simulink model "testing_DM_hby"  (R2023b)
settings: Solver=FixedStepDiscrete  StartTime=0.0  StopTime=inf  FixedStep=0.003  RelTol=1e-3
InitFcn:
  | run('/home/uonaim/matlab_ws/FOOT/joint_calibration.m');
undefined symbols (not defined in the file or in its folder): CAL
libraries: ros2lib x12
(part 1 of 2)
settings Model: Creator=root  LastModifiedBy=root
settings OptimizationCC: EnhancedBackFolding=on  PassReuseOutputArgsAs=Individual arguments  ZeroExternalMemoryAtStartup=off  ZeroInternalMemoryAtStartup=off  MaxStackSize=64  OptimizeBlockOrder=speed  DifferentSizesBufferReuse=on  OptimizationCustomize=off  EfficientTunableParamExpr=on
settings DebuggingCC: ParameterTunabilityLossMsg=error
settings HardwareCC: ProdBitPerLong=64  ProdHWDeviceType=Intel->x86-64 (Linux 64)
settings SFSimCC: MATLABDynamicMemAlloc=off
settings RTWCC: Description=Embedded Coder  SystemTargetFile=ert.tlc  HardwareBoard=Robot Operating System 2 (ROS 2)  TLCOptions="-aInlineSetEventsForThisBaseRateFcn=TLC_FALSE -aSuppressMultiTaskScheduler=TLC_FALSE  -aRateBasedStepFcn=0"  TemplateMakefile=ert_default_tmf  Toolchain=Colcon Tools  TargetLang=C++
settings CodeAppCC: ForceParamTrailComments=on  IgnoreCustomStorageClasses=off  OperatorAnnotations=on  SimulinkDataObjDesc=on  SFDataObjDesc=on  InsertBlockDesc=on
settings ERTTargetCC: CodeInterfacePackaging=C++ class  SupportContinuousTime=on  RootIOFormat=Structure reference

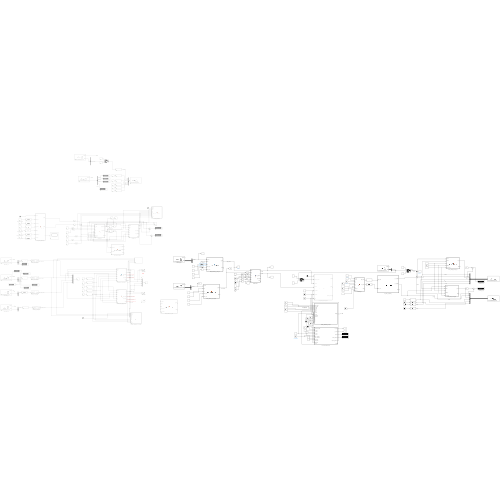
[thumbnail: Simulink's stored preview of the top-level diagram]
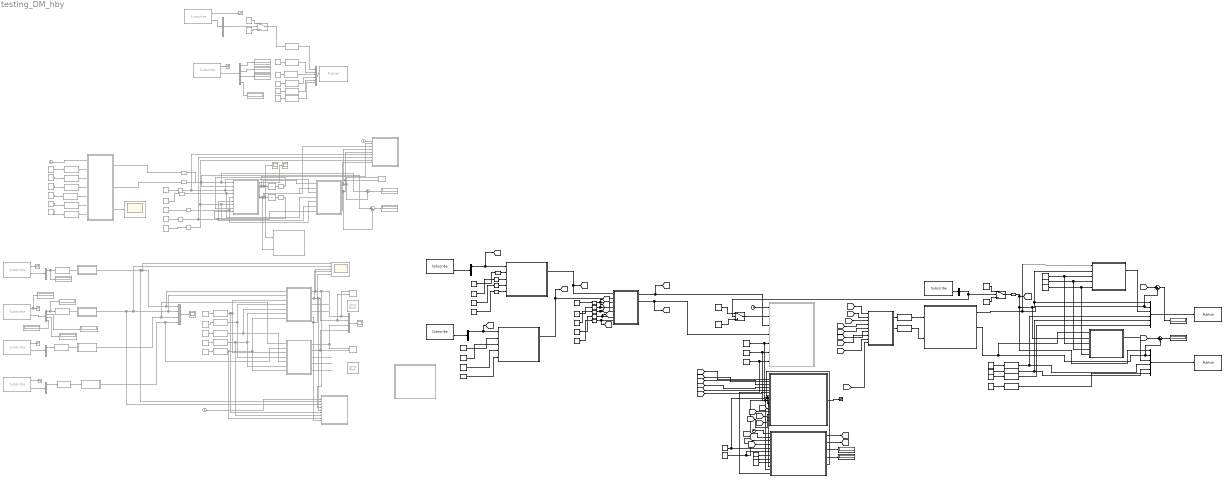
== system testing_DM_hby ==
  note: single(20)
  A : Constant  Value=-0.24
  Alpha Memory : UnitDelay  Commented=on  InitialCondition=CAL.qj0_LA  SampleTime=-1  HasFrameUpgradeWarning=on
  B : Constant  Value=0.24
  Beta Memory : UnitDelay  Commented=on  InitialCondition=CAL.qj0_LB  SampleTime=-1  HasFrameUpgradeWarning=on
  Bus Creator : BusCreator  Commented=on  Inputs=6  OutDataTypeStr=Bus: SL_Bus_custom_msgs_WriteDmMotorMITControl  NonVirtualBus=on
      settings: InheritFromInputs=off
  Bus Creator1 : BusCreator  Inputs=6  OutDataTypeStr=Bus: SL_Bus_custom_msgs_WriteDmMotorMITControl  NonVirtualBus=on
  Bus Creator2 : BusCreator  Inputs=6  OutDataTypeStr=Bus: SL_Bus_custom_msgs_WriteDmMotorMITControl  NonVirtualBus=on
  Bus Selector : BusSelector  Commented=on  OutputSignals=position,velocity,torque,online
  Bus Selector1 : BusSelector  Commented=on  OutputSignals=right_switch
  Bus Selector2 : BusSelector  Commented=on  OutputSignals=position,velocity,torque
  Bus Selector3 : BusSelector  Commented=on  OutputSignals=position,velocity,torque
  Bus Selector4 : BusSelector  Commented=on  OutputSignals=position,velocity,torque,overload
  Bus Selector5 : BusSelector  Commented=on  OutputSignals=position,velocity,torque
  Bus Selector6 : BusSelector  OutputSignals=position,velocity,torque
  Bus Selector7 : BusSelector  OutputSignals=position,velocity,torque
  Bus Selector8 : BusSelector  OutputSignals=right_switch
  Clock : Clock  Commented=on
  Clock1 : Clock  Commented=on
  Clock2 : Clock  Commented=on
  Clock3 : Clock
  Clock4 : Clock
  Constant : Constant  Commented=on
  Constant{1,4..6} (4 alike) : Constant  Commented=on  Value=0
  Constant10 : Constant  Value=CAL.ratio_LA
  Constant11 : Constant  Value=CAL.ratio_LB
  Constant12 : Constant  Value=CAL.qm0_LB
  Constant13 : Constant  Value=CAL.qj0_LB
  Constant14 : Constant  Value=CAL.sign_LB
  Constant15 : Constant  Value=true  OutDataTypeStr=boolean
  Constant16 : Constant  Value=single(0.05)
  Constant17 : Constant  Value=single(0.02)
  Constant18 : Constant  Value=single(20)
  Constant19 : Constant  Value=single(0.035)
  Constant2 : Constant  Commented=on  Value=0.9
  Constant20 : Constant  Value=single(0.1)
  Constant21 : Constant  Value=single(5.0)
  Constant22 : Constant  Value=single(0.003)
  Constant23 : Constant
  Constant24 : Constant  Value=0
  Constant25 : Constant  Value=single(0.5)
  Constant26 : Constant  Value=3.3
  Constant27 : Constant  Value=0.09
  Constant29 : Constant  Value=single(0.003)
  Constant3 : Constant  Commented=on  Value=0.1
  Constant30 : Constant  Value=single(8.0)
  Constant31 : Constant  Value=single(0.5)
  Constant32 : Constant  Value=false  OutDataTypeStr=boolean
  Constant7 : Constant  Value=CAL.qm0_LA
  Constant8 : Constant  Value=CAL.qj0_LA
  Constant9 : Constant  Value=CAL.sign_LA
  Data Type Conversion : DataTypeConversion  Commented=on  OutDataTypeStr=uint8  SaturateOnIntegerOverflow=off  RndMeth=Floor
  Data Type Conversion{1..29} (29 alike) : DataTypeConversion  Commented=on  OutDataTypeStr=single  SaturateOnIntegerOverflow=off  RndMeth=Floor
  Data Type Conversion{30..40,42,46..48} (15 alike) : DataTypeConversion  OutDataTypeStr=single  SaturateOnIntegerOverflow=off  RndMeth=Floor
  Data Type Conversion41 : DataTypeConversion  OutDataTypeStr=uint8  SaturateOnIntegerOverflow=off  RndMeth=Floor
  Display{,1..11} (12 alike) : Display  Commented=on
  Display12 : Display
  Display13 : Display
  FiveBar_Animation : MATLAB Function  Commented=on  TreatAsAtomicUnit=on
  FiveBar_Animation_Compare : MATLAB Function  TreatAsAtomicUnit=on
  FiveBar_Animation_Left_Actual : MATLAB Function  Commented=on  TreatAsAtomicUnit=on
  FiveBar_FK : MATLAB Function  Commented=on  TreatAsAtomicUnit=on
  FiveBar_FK1 : MATLAB Function  TreatAsAtomicUnit=on
  FiveBar_FK_Left_Actual : MATLAB Function  Commented=on  TreatAsAtomicUnit=on
  FiveBar_FK_Right_Actual : MATLAB Function  Commented=on  TreatAsAtomicUnit=on
  FiveBar_IK : MATLAB Function  Commented=on  TreatAsAtomicUnit=on
  FiveBar_IK1 : MATLAB Function  TreatAsAtomicUnit=on
  Foot_Home_Then_Sine : MATLAB Function  TreatAsAtomicUnit=on
  Foot_Sine_Trajectory : MATLAB Function  Commented=on  TreatAsAtomicUnit=on
  Foot_Sine_Trajectory_HW : MATLAB Function  Commented=on  TreatAsAtomicUnit=on
  L{1,4,6,9} (4 alike) : Constant  Commented=on  Value=0.0804
  L10 : Constant  Commented=on  Value=0.07
  L11 : Constant  Value=0.0804
  L12 : Constant  Value=0.12
  L13 : Constant  Value=0.12
  L14 : Constant  Value=0.0804
  L15 : Constant  Value=0.07
  L{2..3,7..8} (4 alike) : Constant  Commented=on  Value=0.12
  L5 : Constant  Commented=on  Value=0.07
  Lamp : LampBlock  Commented=on  LabelPosition=Hide  Icon=Check3
  Lamp1 : LampBlock  Commented=on  LabelPosition=Hide
  Left_Joint_To_Motor : MATLAB Function  Commented=on  TreatAsAtomicUnit=on
  Left_Joint_To_Motor_L : MATLAB Function  TreatAsAtomicUnit=on
  Motor_Position_To_Joint : MATLAB Function  Commented=on  TreatAsAtomicUnit=on
  Motor_Position_To_Joint_LA : MATLAB Function  TreatAsAtomicUnit=on
  Motor_Position_To_Joint_LB : MATLAB Function  TreatAsAtomicUnit=on
  Motor_Target_Velocity_LA : MATLAB Function  TreatAsAtomicUnit=on
  Motor_Target_Velocity_LB : MATLAB Function  TreatAsAtomicUnit=on
  Motor_To_Joint_LA : Subsystem  Commented=on
  Motor_To_Joint_LB : Subsystem  Commented=on
  Motor_To_Joint_RA : Subsystem  Commented=on
  Motor_To_Joint_RB : Subsystem  Commented=on
  Mux : Mux  Commented=on
  Mux1 : Mux  Commented=on
  Publish : ros2lib/Publish  Commented=on  topicSource=Select from ROS network  topic=/ecat/sn2228252/app4/write  messageType=custom_msgs/WriteDmMotorMITControl  QOSHistory=Keep last  QOSDepth=1  QOSReliability=Best effort  QOSDurability=Volatile
  Publish1 : ros2lib/Publish  topicSource=Select from ROS network  topic=/ecat/sn2228252/app2/write  messageType=custom_msgs/WriteDmMotorMITControl  QOSHistory=Keep last  QOSDepth=1  QOSReliability=Best effort  QOSDurability=Volatile
  Publish2 : ros2lib/Publish  topicSource=Select from ROS network  topic=/ecat/sn2228252/app3/write  messageType=custom_msgs/WriteDmMotorMITControl  QOSHistory=Keep last  QOSDepth=1  QOSReliability=Best effort  QOSDurability=Volatile
  Scope{,1..4} (5 alike) : Scope  Commented=on
  Scope5 : Scope  Commented=on  NumInputPorts=5
  Subscribe : ros2lib/Subscribe  Commented=on  topicSource=Select from ROS network  topic=/ecat/sn2228252/app4/read  messageType=custom_msgs/ReadDmMotor  sampleTime=-1  QOSHistory=Keep last  QOSDepth=1  QOSReliability=Best effort  QOSDurability=Volatile
  Subscribe1 : ros2lib/Subscribe  Commented=on  topicSource=Select from ROS network  topic=/ecat/sn2228252/app1/read  messageType=custom_msgs/ReadDJIRC  sampleTime=-1  QOSHistory=Keep last  QOSDepth=1  QOSReliability=Best effort  QOSDurability=Volatile
  Subscribe2 : ros2lib/Subscribe  Commented=on  topicSource=Select from ROS network  topic=/ecat/sn2228252/app3/read  messageType=custom_msgs/ReadDmMotor  sampleTime=-1  QOSHistory=Keep last  QOSDepth=1  QOSReliability=Best effort  QOSDurability=Volatile
  Subscribe3 : ros2lib/Subscribe  topicSource=Select from ROS network  topic=/ecat/sn2228252/app3/read  messageType=custom_msgs/ReadDmMotor  sampleTime=-1  QOSHistory=Keep last  QOSDepth=1  QOSReliability=Best effort  QOSDurability=Volatile
  Subscribe4 : ros2lib/Subscribe  topicSource=Select from ROS network  topic=/ecat/sn2228252/app1/read  messageType=custom_msgs/ReadDJIRC  sampleTime=-1  QOSHistory=Keep last  QOSDepth=1  QOSReliability=Best effort  QOSDurability=Volatile
  Subscribe_LA : ros2lib/Subscribe  Commented=on  topicSource=Select from ROS network  topic=/ecat/sn2228252/app2/read  messageType=custom_msgs/ReadDmMotor  sampleTime=-1  QOSHistory=Keep last  QOSDepth=1  QOSReliability=Best effort  QOSDurability=Volatile
  Subscribe_LA1 : ros2lib/Subscribe  topicSource=Select from ROS network  topic=/ecat/sn2228252/app2/read  messageType=custom_msgs/ReadDmMotor  sampleTime=-1  QOSHistory=Keep last  QOSDepth=1  QOSReliability=Best effort  QOSDurability=Volatile
  Subscribe_RA : ros2lib/Subscribe  Commented=on  topicSource=Select from ROS network  topic=/ecat/sn2228252/app5/read  messageType=custom_msgs/ReadDmMotor  sampleTime=-1  QOSHistory=Keep last  QOSDepth=1  QOSReliability=Best effort  QOSDurability=Volatile
  Subscribe_RB : ros2lib/Subscribe  Commented=on  topicSource=Select from ROS network  topic=/ecat/sn2228252/app6/read  messageType=custom_msgs/ReadDmMotor  sampleTime=-1  QOSHistory=Keep last  QOSDepth=1  QOSReliability=Best effort  QOSDurability=Volatile
  Sum : Sum  Inputs=|+-
  Sum1 : Sum  Inputs=|+-
  Switch : Switch  Commented=on  Criteria=u2 > Threshold  Threshold=2  SaturateOnIntegerOverflow=off  InputSameDT=off
  Switch1 : Switch  Criteria=u2 > Threshold  Threshold=2  SaturateOnIntegerOverflow=off  InputSameDT=off
  Switch2 : Switch  Criteria=u2 > Threshold  Threshold=2  SaturateOnIntegerOverflow=off  InputSameDT=off
  Terminator{,1..5} (6 alike) : Terminator  Commented=on
  Terminator6 : Terminator
  Trajectory_Amplitude : Constant  Commented=on  Value=0.01
  Trajectory_Enable : Constant  Commented=on
  Trajectory_Period : Constant  Commented=on  Value=10
  Trajectory_Width : Constant  Commented=on  Value=0.02
  X Error : Sum  Commented=on  Inputs=|+-
  XY Graph : Record  Commented=on  FileSettingsInternal="{\"entries\":[{\"content\":{\"excelSettings\":{\"content\":{},\"type\":\"Streamout.ExcelSettings\"}},\"type\":\"Streamout.FileSettingStorage\",\"uuid\":\"\"}],\"packageUris\":[\"http:\\/\\/schema.mathworks.com\\/mf0\\/streamout_blocks\\/R2020a\"],\"version\":\"1.0\"}"  Layout=[1 1]  SignalsInternal="{\"entries\":[{\"content\":{\"signals\":[{\"content\":{\"blockPath\":[],\"dimensions\":[1],\"domain\":\"\",\"lineColor\":\"#a2142f\",\"port\":1,\"sid\":[\"\"],\"signalID\":1,\"signalName\":\"FiveBar_FK:1\"},\"type\":\"RecordBlkView.Signal\",\"uuid\":\"\"},{\"content\":{\"blockPath\":[],\"dimensions\":[1],\"domain\":\"\",\"lineColor\":\"#139fff\",\"port\":2,\"sid\":[\"\"],\"signalID\":2,\"signalName\":\"FiveBar_FK:2\"},\"type\":\"RecordBlkView.Signal\",\"uuid\":\"\"}]},\"type\":\"RecordBlkView.InputSignals\",\"uuid\":\"\"}],\"packageUris\":[\"http:\\/\\/schema.mathworks.com\\/mf0\\/streamout_blocks\\/R2020a\"],\"version\":\"1.0\"}"  VisualizationBindings="{\"xyplotplugin\":{\"info\":[{\"series\":[],\"subplotID\":1}]}}"  CompatibilityTag=XY
  XY Graph1 : Record  Commented=on  FileSettingsInternal="{\"entries\":[{\"content\":{\"excelSettings\":{\"content\":{},\"type\":\"Streamout.ExcelSettings\"}},\"type\":\"Streamout.FileSettingStorage\",\"uuid\":\"\"}],\"packageUris\":[\"http:\\/\\/schema.mathworks.com\\/mf0\\/streamout_blocks\\/R2020a\"],\"version\":\"1.0\"}"  Layout=[1 1]  SignalsInternal="{\"entries\":[{\"content\":{},\"type\":\"RecordBlkView.InputSignals\",\"uuid\":\"\"}],\"packageUris\":[\"http:\\/\\/schema.mathworks.com\\/mf0\\/streamout_blocks\\/R2020a\"],\"version\":\"1.0\"}"  VisualizationBindings="{\"xyplotplugin\":{\"info\":[{\"series\":[],\"subplotID\":1}]}}"  CompatibilityTag=XY
  XY Graph2 : Record  Commented=on  FileSettingsInternal="{\"entries\":[{\"content\":{\"excelSettings\":{\"content\":{},\"type\":\"Streamout.ExcelSettings\"}},\"type\":\"Streamout.FileSettingStorage\",\"uuid\":\"\"}],\"packageUris\":[\"http:\\/\\/schema.mathworks.com\\/mf0\\/streamout_blocks\\/R2020a\"],\"version\":\"1.0\"}"  Layout=[1 1]  SignalsInternal="{\"entries\":[{\"content\":{},\"type\":\"RecordBlkView.InputSignals\",\"uuid\":\"\"}],\"packageUris\":[\"http:\\/\\/schema.mathworks.com\\/mf0\\/streamout_blocks\\/R2020a\"],\"version\":\"1.0\"}"  VisualizationBindings="{\"xyplotplugin\":{\"info\":[{\"series\":[],\"subplotID\":1}]}}"  CompatibilityTag=XY
  X_Center : Constant  Commented=on  Value=0.035
  Y Error : Sum  Commented=on  Inputs=|+-
  Y_Center : Constant  Commented=on  Value=0.12
  position_err_A : Display
  position_err_B : Display
  wires:
  Subscribe/1 -> Terminator/1
  Subscribe/2 -> Bus Selector/1
  Bus Selector/4 -> Display/1  "<online>"
  Bus Selector/1 -> Display3/1  "<position>"
  Bus Selector/2 -> Display1/1  "<velocity>"
  Bus Selector/3 -> Display2/1  "<torque>"
  Bus Creator/1 -> Publish/1
  Constant1/1 -> Data Type Conversion1/1
  Constant3/1 -> Data Type Conversion4/1
  Constant4/1 -> Data Type Conversion3/1
  Constant2/1 -> Data Type Conversion2/1
  Data Type Conversion/1 -> Bus Creator/1  "enable"
  Data Type Conversion1/1 -> Bus Creator/2  "p_des"
  Data Type Conversion2/1 -> Bus Creator/3  "v_des"
  Data Type Conversion3/1 -> Bus Creator/4  "kp"
  Data Type Conversion4/1 -> Bus Creator/5  "kd"
  Constant5/1 -> Data Type Conversion5/1
  Data Type Conversion5/1 -> Bus Creator/6  "torque"
  Constant/1 -> Switch/1
  Switch/1 -> Data Type Conversion/1
  Subscribe1/1 -> Terminator1/1
  Subscribe1/2 -> Bus Selector1/1
  Bus Selector1/1 -> Switch/2  "<right_switch>"
  Constant6/1 -> Switch/3
  FiveBar_IK/1(alpha_cmd) -> FiveBar_Animation/2(alpha), FiveBar_FK/1(alpha), Left_Joint_To_Motor/1(alpha_cmd), Scope1/1, Alpha Memory/1
  Alpha Memory/1 -> Data Type Conversion6/1
  FiveBar_IK/2(beta_cmd) -> Left_Joint_To_Motor/2(beta_cmd), FiveBar_Animation/3(beta), Beta Memory/1, FiveBar_FK/2(beta), Scope2/1
  Beta Memory/1 -> Data Type Conversion7/1
  L2/1 -> Data Type Conversion11/1
  L3/1 -> Data Type Conversion12/1
  L4/1 -> Data Type Conversion13/1
  L5/1 -> Data Type Conversion14/1
  L1/1 -> Data Type Conversion10/1
  FiveBar_FK/1(x) -> FiveBar_Animation/4(xB), X Error/2, XY Graph/1
  FiveBar_FK/2(y) -> XY Graph/2, FiveBar_Animation/5(yB), Y Error/2
  X Error/1 -> Display4/1
  Y Error/1 -> Display5/1
  Data Type Conversion6/1 -> FiveBar_IK/8(alpha_ref)
  Data Type Conversion7/1 -> FiveBar_IK/9(beta_ref)
  Data Type Conversion8/1 -> X Error/1, FiveBar_IK/1(x_cmd)
  Data Type Conversion9/1 -> Y Error/1, FiveBar_IK/2(y_cmd)
  Data Type Conversion10/1 -> FiveBar_Animation/6(L1), FiveBar_FK/3(L1), FiveBar_IK/3(L1)
  Data Type Conversion11/1 -> FiveBar_FK/4(L2), FiveBar_IK/4(L2)
  Data Type Conversion12/1 -> FiveBar_IK/5(L3), FiveBar_FK/5(L3)
  Data Type Conversion13/1 -> FiveBar_Animation/7(L4), FiveBar_IK/6(L4), FiveBar_FK/6(L4)
  Data Type Conversion14/1 -> FiveBar_Animation/8(L5), FiveBar_FK/7(L5), FiveBar_IK/7(L5)
  FiveBar_FK/5(valid) -> FiveBar_Animation/9(valid)
  Trajectory_Enable/1 -> Data Type Conversion16/1
  Clock/1 -> Foot_Sine_Trajectory/1(time_in)
  Data Type Conversion16/1 -> Foot_Sine_Trajectory/2(enable_in)
  X_Center/1 -> Data Type Conversion17/1
  Y_Center/1 -> Data Type Conversion18/1
  Data Type Conversion17/1 -> Foot_Sine_Trajectory/3(x_center_in)
  Data Type Conversion18/1 -> Foot_Sine_Trajectory/4(y_center_in)
  Trajectory_Width/1 -> Data Type Conversion19/1
  Data Type Conversion19/1 -> Foot_Sine_Trajectory/5(width_in)
  Trajectory_Amplitude/1 -> Data Type Conversion20/1
  Data Type Conversion20/1 -> Foot_Sine_Trajectory/6(amplitude_in)
  Trajectory_Period/1 -> Data Type Conversion21/1
  Data Type Conversion21/1 -> Foot_Sine_Trajectory/7(period_in)
  Foot_Sine_Trajectory/1(x_cmd) -> Data Type Conversion8/1
  Foot_Sine_Trajectory/2(y_cmd) -> Data Type Conversion9/1
  Foot_Sine_Trajectory/3(s) -> Scope/1
  Clock1/1 -> FiveBar_Animation/1(time_in)
  Subscribe_LA/2 -> Bus Selector2/1
  Bus Selector2/1 -> Display11/1, Data Type Conversion15/1  "<position>"
  Subscribe_LA/1 -> Terminator2/1
  Subscribe_RA/2 -> Bus Selector3/1
  Subscribe_RB/2 -> Bus Selector5/1
  Subscribe2/2 -> Bus Selector4/1
  Subscribe2/1 -> Display6/1, Terminator3/1
  Subscribe_RA/1 -> Terminator4/1
  Subscribe_RB/1 -> Terminator5/1
  Bus Selector3/1 -> Data Type Conversion23/1  "<position>"
  Bus Selector5/1 -> Data Type Conversion24/1  "<position>"
  Data Type Conversion15/1 -> Motor_To_Joint_LA/1(q_motor)
  Data Type Conversion22/1 -> Motor_To_Joint_LB/1(q_motor)
  Data Type Conversion23/1 -> Motor_To_Joint_RA/1(q_motor)
  Data Type Conversion24/1 -> Motor_To_Joint_RB/1(q_motor)
  Motor_To_Joint_LA/1(q_joint) -> FiveBar_Animation_Left_Actual/2(alpha), Scope5/1, FiveBar_FK_Left_Actual/1(alpha), Mux/1  "alpha_left_meas"
  Motor_To_Joint_LB/1(q_joint) -> FiveBar_Animation_Left_Actual/3(beta), Scope5/2, FiveBar_FK_Left_Actual/2(beta), Mux/2  "beta_left_meas"
  Motor_To_Joint_RA/1(q_joint) -> FiveBar_FK_Right_Actual/1(alpha), Mux/3  "alpha_right_meas"
  Motor_To_Joint_RB/1(q_joint) -> FiveBar_FK_Right_Actual/2(beta), Mux/4  "beta_right_meas"
  Mux/1 -> Scope3/1
  L6/1 -> Data Type Conversion25/1
  Data Type Conversion25/1 -> FiveBar_Animation_Left_Actual/6(L1), FiveBar_FK_Right_Actual/3(L1), FiveBar_FK_Left_Actual/3(L1)
  L7/1 -> Data Type Conversion26/1
  Data Type Conversion26/1 -> FiveBar_FK_Left_Actual/4(L2), FiveBar_FK_Right_Actual/4(L2)
  L8/1 -> Data Type Conversion27/1
  Data Type Conversion27/1 -> FiveBar_FK_Right_Actual/5(L3), FiveBar_FK_Left_Actual/5(L3)
  L9/1 -> Data Type Conversion28/1
  L10/1 -> Data Type Conversion29/1
  Data Type Conversion29/1 -> FiveBar_Animation_Left_Actual/8(L5), FiveBar_FK_Left_Actual/7(L5), FiveBar_FK_Right_Actual/7(L5)
  FiveBar_FK_Left_Actual/1(x) -> Scope5/3, FiveBar_Animation_Left_Actual/4(xB), XY Graph1/1, Mux1/1  "x_left_actual"
  FiveBar_FK_Left_Actual/2(y) -> Scope5/4, FiveBar_Animation_Left_Actual/5(yB), XY Graph1/2, Mux1/2  "y_left_actual"
  FiveBar_FK_Left_Actual/3(leg_length) -> ?  "leg_length_left_actual"
  FiveBar_FK_Left_Actual/4(leg_angle) -> ?  "leg_angle_left_actual"
  FiveBar_FK_Left_Actual/5(valid) -> Scope5/5, FiveBar_Animation_Left_Actual/9(valid)  "fk_valid_left"
  FiveBar_FK_Right_Actual/1(x) -> XY Graph2/1, Mux1/3  "x_right_actual"
  FiveBar_FK_Right_Actual/2(y) -> XY Graph2/2, Mux1/4  "y_right_actual"
  FiveBar_FK_Right_Actual/3(leg_length) -> ?  "leg_length_right_actual"
  FiveBar_FK_Right_Actual/4(leg_angle) -> ?  "leg_angle_right_actual"
  FiveBar_FK_Right_Actual/5(valid) -> ?  "fk_valid_right"
  Mux1/1 -> Scope4/1
  Clock2/1 -> FiveBar_Animation_Left_Actual/1(time_in)
  Data Type Conversion28/1 -> FiveBar_Animation_Left_Actual/7(L4), FiveBar_FK_Right_Actual/6(L4), FiveBar_FK_Left_Actual/6(L4)
  Bus Selector4/1 -> Data Type Conversion22/1, Display7/1  "<position>"
  Bus Selector4/2 -> Display8/1  "<velocity>"
  Bus Selector4/3 -> Display9/1  "<torque>"
  Bus Selector4/4 -> Display10/1  "<overload>"
  Subscribe_LA1/2 -> Bus Selector6/1
  Bus Selector6/1 -> [actual_pos_A], Motor_Position_To_Joint_LA/1(q_motor)  "<position>"
  Constant7/1 -> Data Type Conversion35/1
  Constant8/1 -> Data Type Conversion36/1
  Constant9/1 -> Data Type Conversion37/1
  Constant10/1 -> Data Type Conversion38/1
  Subscribe3/2 -> Bus Selector7/1
  Bus Selector7/1 -> [actual_pos_B], Motor_Position_To_Joint_LB/1(q_motor)  "<position>"
  Constant13/1 -> Motor_Position_To_Joint_LB/3(qj0)
  Constant12/1 -> Motor_Position_To_Joint_LB/2(qm0)
  Constant14/1 -> Motor_Position_To_Joint_LB/4(motor_sign)
  Constant11/1 -> Motor_Position_To_Joint_LB/5(motor_ratio)
  Motor_Position_To_Joint_LA/1(q_joint) -> [alpha_actual], FiveBar_FK1/1(alpha)  "alpha_actual"
  Motor_Position_To_Joint_LB/1(q_joint) -> FiveBar_FK1/2(beta), [beta_actual]  "beta_actual"
  L15/1 -> Data Type Conversion34/1
  L14/1 -> Data Type Conversion33/1
  L11/1 -> Data Type Conversion30/1
  L12/1 -> Data Type Conversion31/1
  L13/1 -> Data Type Conversion32/1
  Data Type Conversion30/1 -> [L1], FiveBar_FK1/3(L1)
  Data Type Conversion31/1 -> [L2], FiveBar_FK1/4(L2)
  Data Type Conversion33/1 -> [L4], FiveBar_FK1/6(L4)
  Data Type Conversion34/1 -> [L5], FiveBar_FK1/7(L5)
  Data Type Conversion35/1 -> Motor_Position_To_Joint_LA/2(qm0)
  Data Type Conversion36/1 -> Motor_Position_To_Joint_LA/3(qj0)
  Data Type Conversion37/1 -> Motor_Position_To_Joint_LA/4(motor_sign)
  Data Type Conversion38/1 -> Motor_Position_To_Joint_LA/5(motor_ratio)
  FiveBar_FK1/1(x) -> [x_actual], Foot_Sine_Trajectory_HW/3(x_actual)  "x_actual"
  FiveBar_FK1/2(y) -> [y_actual], Foot_Sine_Trajectory_HW/4(y_actual)  "y_actual"
  Clock3/1 -> Foot_Sine_Trajectory_HW/1(t)
  Constant16/1 -> Foot_Home_Then_Sine/10(path_width), FiveBar_Animation_Compare/10(path_width), Foot_Sine_Trajectory_HW/5(path_width)
  Constant17/1 -> Foot_Home_Then_Sine/11(amplitude), FiveBar_Animation_Compare/11(amplitude), Foot_Sine_Trajectory_HW/6(amplitude)
  Constant18/1 -> Foot_Home_Then_Sine/12(period), Foot_Sine_Trajectory_HW/7(period)
  [L1] -> FiveBar_IK1/3(L1)
  [L2] -> FiveBar_IK1/4(L2)
  [L3] -> FiveBar_IK1/5(L3)
  [L4] -> FiveBar_IK1/6(L4)
  [L5] -> FiveBar_IK1/7(L5)
  Data Type Conversion32/1 -> [L3], FiveBar_FK1/5(L3)
  FiveBar_IK1/1(alpha_cmd) -> Data Type Conversion39/1
  FiveBar_IK1/2(beta_cmd) -> Data Type Conversion40/1
  [alpha_actual] -> FiveBar_IK1/8(alpha_ref)
  [beta_actual] -> FiveBar_IK1/9(beta_ref)
  Data Type Conversion39/1 -> Left_Joint_To_Motor_L/1(alpha_cmd)
  Data Type Conversion40/1 -> Left_Joint_To_Motor_L/2(beta_cmd)
  Left_Joint_To_Motor_L/1(p_LA_target) -> Motor_Target_Velocity_LA/1(p_cmd), Sum/2, Bus Creator1/2  "p_des"
  Bus Creator1/1 -> Publish1/1
  Constant23/1 -> Switch1/1
  Constant24/1 -> Switch1/3
  Subscribe4/2 -> Bus Selector8/1
  Bus Selector8/1 -> Switch2/2, Switch1/2  "<right_switch>"
  Switch1/1 -> Data Type Conversion41/1  "enable"
  Bus Creator2/1 -> Publish2/1
  Constant26/1 -> Data Type Conversion46/1
  Constant27/1 -> Data Type Conversion47/1
  A/1 -> Data Type Conversion48/1
  Left_Joint_To_Motor_L/2(p_LB_target) -> Motor_Target_Velocity_LB/1(p_cmd), Sum1/2, Bus Creator2/2  "p_des"
  Data Type Conversion46/1 -> Bus Creator1/4, Bus Creator2/4  "kp"
  Data Type Conversion47/1 -> Bus Creator1/5, Bus Creator2/5  "kd"
  Data Type Conversion48/1 -> Bus Creator1/6  "torque"
  Constant29/1 -> Motor_Target_Velocity_LB/3(Ts), Motor_Target_Velocity_LA/3(Ts)
  Constant30/1 -> Motor_Target_Velocity_LB/4(cutoff_hz), Motor_Target_Velocity_LA/4(cutoff_hz)
  Constant31/1 -> Motor_Target_Velocity_LB/5(max_velocity), Motor_Target_Velocity_LA/5(max_velocity)
  Motor_Target_Velocity_LA/1(v_des) -> Bus Creator1/3  "v_des"
  Motor_Target_Velocity_LB/1(v_des) -> Bus Creator2/3  "v_des"
  Switch2/1 -> Foot_Sine_Trajectory_HW/2(trajectory_enable)
  Constant15/1 -> Switch2/1
  Constant32/1 -> Switch2/3
  [alpha_actual] -> FiveBar_Animation_Compare/1(alpha_actual)
  [beta_actual] -> FiveBar_Animation_Compare/2(beta_actual)
  [x_actual] -> FiveBar_Animation_Compare/3(x_actual)
  [y_actual] -> FiveBar_Animation_Compare/4(y_actual)
  [x_cmd2] -> FiveBar_Animation_Compare/5(x_cmd)
  [y_cmd2] -> FiveBar_Animation_Compare/6(y_cmd)
  [L2] -> FiveBar_Animation_Compare/13(L2)
  [L1] -> FiveBar_Animation_Compare/12(L1)
  [L3] -> FiveBar_Animation_Compare/14(L3)
  [L4] -> FiveBar_Animation_Compare/15(L4)
  [L5] -> FiveBar_Animation_Compare/16(L5)
  FiveBar_Animation_Compare/1(dummy) -> Terminator6/1
  Data Type Conversion41/1 -> [enable], Bus Creator2/1, Motor_Target_Velocity_LB/2(enable), Motor_Target_Velocity_LA/2(enable), Bus Creator1/1  "enable"
  [x_actual] -> Foot_Home_Then_Sine/3(x_actual)
  Constant19/1 -> FiveBar_Animation_Compare/8(x_home), Foot_Home_Then_Sine/5(x_home)
  Clock4/1 -> Foot_Home_Then_Sine/1(t)
  [y_actual] -> Foot_Home_Then_Sine/4(y_actual)
  Constant21/1 -> Foot_Home_Then_Sine/7(home_duration)
  Constant20/1 -> FiveBar_Animation_Compare/9(y_home), Foot_Home_Then_Sine/6(y_home)
  [enable] -> Foot_Home_Then_Sine/2(sequence_enable)
  Constant22/1 -> Foot_Home_Then_Sine/8(home_tolerance)
  Constant25/1 -> Foot_Home_Then_Sine/9(settle_time)
  Foot_Home_Then_Sine/2(y_cmd) -> [y_cmd2]
  Foot_Home_Then_Sine/1(x_cmd) -> [x_cmd2]
  [x_cmd2] -> FiveBar_IK1/1(x_cmd)
  [y_cmd2] -> FiveBar_IK1/2(y_cmd)
  Foot_Home_Then_Sine/3(phase) -> Display12/1
  Foot_Home_Then_Sine/4(home_reached) -> Display13/1
  Foot_Home_Then_Sine/5(trajectory_active) -> FiveBar_Animation_Compare/7(phase)
  B/1 -> Data Type Conversion42/1
  Data Type Conversion42/1 -> Bus Creator2/6  "torque"
  [actual_pos_A] -> Sum/1
  Sum/1 -> position_err_A/1
  [actual_pos_B] -> Sum1/1
  Sum1/1 -> position_err_B/1

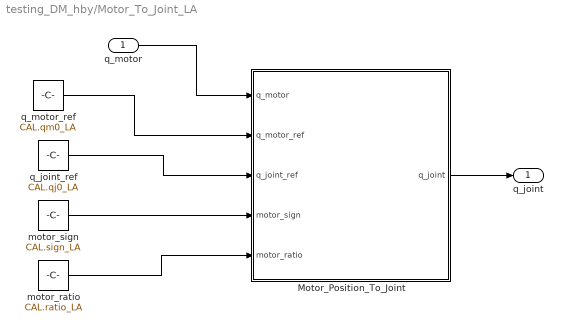
== system testing_DM_hby/Motor_To_Joint_LA ==
  q_motor : Inport
  Motor_Position_To_Joint : MATLAB Function  TreatAsAtomicUnit=on
  motor_ratio : Constant  Value=CAL.ratio_LA
  motor_sign : Constant  Value=CAL.sign_LA
  q_joint_ref : Constant  Value=CAL.qj0_LA
  q_motor_ref : Constant  Value=CAL.qm0_LA
  q_joint : Outport
  wires:
  q_motor/1 -> Motor_Position_To_Joint/1(q_motor)
  q_motor_ref/1 -> Motor_Position_To_Joint/2(q_motor_ref)
  q_joint_ref/1 -> Motor_Position_To_Joint/3(q_joint_ref)
  motor_sign/1 -> Motor_Position_To_Joint/4(motor_sign)
  motor_ratio/1 -> Motor_Position_To_Joint/5(motor_ratio)
  Motor_Position_To_Joint/1(q_joint) -> q_joint/1

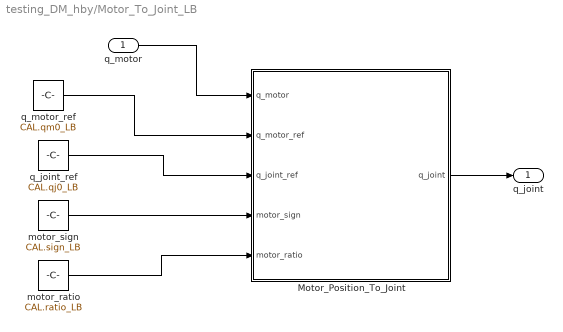
== system testing_DM_hby/Motor_To_Joint_LB ==
  q_motor : Inport
  Motor_Position_To_Joint : MATLAB Function  TreatAsAtomicUnit=on
  motor_ratio : Constant  Value=CAL.ratio_LB
  motor_sign : Constant  Value=CAL.sign_LB
  q_joint_ref : Constant  Value=CAL.qj0_LB
  q_motor_ref : Constant  Value=CAL.qm0_LB
  q_joint : Outport
  wires:
  q_motor/1 -> Motor_Position_To_Joint/1(q_motor)
  q_motor_ref/1 -> Motor_Position_To_Joint/2(q_motor_ref)
  q_joint_ref/1 -> Motor_Position_To_Joint/3(q_joint_ref)
  motor_sign/1 -> Motor_Position_To_Joint/4(motor_sign)
  motor_ratio/1 -> Motor_Position_To_Joint/5(motor_ratio)
  Motor_Position_To_Joint/1(q_joint) -> q_joint/1

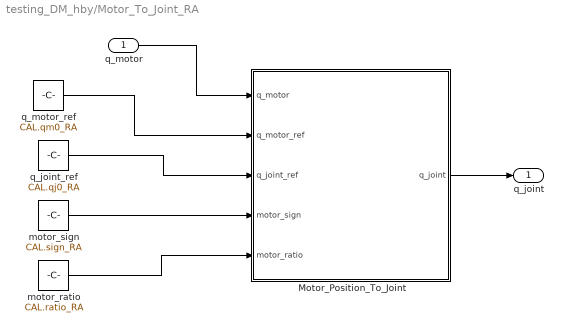
== system testing_DM_hby/Motor_To_Joint_RA ==
  q_motor : Inport
  Motor_Position_To_Joint : MATLAB Function  TreatAsAtomicUnit=on
  motor_ratio : Constant  Value=CAL.ratio_RA
  motor_sign : Constant  Value=CAL.sign_RA
  q_joint_ref : Constant  Value=CAL.qj0_RA
  q_motor_ref : Constant  Value=CAL.qm0_RA
  q_joint : Outport
  wires:
  q_motor/1 -> Motor_Position_To_Joint/1(q_motor)
  q_motor_ref/1 -> Motor_Position_To_Joint/2(q_motor_ref)
  q_joint_ref/1 -> Motor_Position_To_Joint/3(q_joint_ref)
  motor_sign/1 -> Motor_Position_To_Joint/4(motor_sign)
  motor_ratio/1 -> Motor_Position_To_Joint/5(motor_ratio)
  Motor_Position_To_Joint/1(q_joint) -> q_joint/1

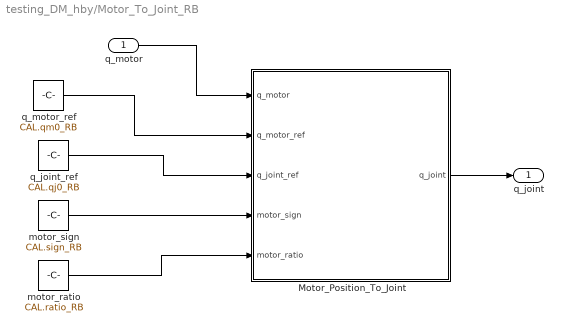
== system testing_DM_hby/Motor_To_Joint_RB ==
  q_motor : Inport
  Motor_Position_To_Joint : MATLAB Function  TreatAsAtomicUnit=on
  motor_ratio : Constant  Value=CAL.ratio_RB
  motor_sign : Constant  Value=CAL.sign_RB
  q_joint_ref : Constant  Value=CAL.qj0_RB
  q_motor_ref : Constant  Value=CAL.qm0_RB
  q_joint : Outport
  wires:
  q_motor/1 -> Motor_Position_To_Joint/1(q_motor)
  q_motor_ref/1 -> Motor_Position_To_Joint/2(q_motor_ref)
  q_joint_ref/1 -> Motor_Position_To_Joint/3(q_joint_ref)
  motor_sign/1 -> Motor_Position_To_Joint/4(motor_sign)
  motor_ratio/1 -> Motor_Position_To_Joint/5(motor_ratio)
  Motor_Position_To_Joint/1(q_joint) -> q_joint/1

== matlab function testing_DM_hby/Motor_To_Joint_LB/Motor_Position_To_Joint ==
  data: q_motor input; q_joint output; q_motor_ref input; q_joint_ref input; motor_sign input; motor_ratio input
function q_joint = motor_position_to_joint( ...
    q_motor, q_motor_ref, q_joint_ref, ...
    motor_sign, motor_ratio)
%#codegen
%
% 电机位置反馈转换为运动学关节角
%
% q_motor      当前电机位置反馈，rad
% q_motor_ref  标定参考姿态下的电机位置，rad
% q_joint_ref  标定参考姿态下的模型关节角，rad
% motor_sign   +1 或 -1
% motor_ratio  电机角变化/关节角变化

qm = single(q_motor);
qm0 = single(q_motor_ref);
qj0 = single(q_joint_ref);
sgn = single(motor_sign);
ratio = single(motor_ratio);

q_joint = qj0;

if abs(ratio) > single(1.0e-6)
    q_joint = qj0 + ...
        sgn * (qm - qm0) / ratio;
end

end

== matlab function testing_DM_hby/Motor_To_Joint_RA/Motor_Position_To_Joint ==
  data: q_motor input; q_joint output; q_motor_ref input; q_joint_ref input; motor_sign input; motor_ratio input
function q_joint = motor_position_to_joint( ...
    q_motor, q_motor_ref, q_joint_ref, ...
    motor_sign, motor_ratio)
%#codegen
%
% 电机位置反馈转换为运动学关节角
%
% q_motor      当前电机位置反馈，rad
% q_motor_ref  标定参考姿态下的电机位置，rad
% q_joint_ref  标定参考姿态下的模型关节角，rad
% motor_sign   +1 或 -1
% motor_ratio  电机角变化/关节角变化

qm = single(q_motor);
qm0 = single(q_motor_ref);
qj0 = single(q_joint_ref);
sgn = single(motor_sign);
ratio = single(motor_ratio);

q_joint = qj0;

if abs(ratio) > single(1.0e-6)
    q_joint = qj0 + ...
        sgn * (qm - qm0) / ratio;
end

end

== matlab function testing_DM_hby/Motor_To_Joint_RB/Motor_Position_To_Joint ==
  data: q_motor input; q_joint output; q_motor_ref input; q_joint_ref input; motor_sign input; motor_ratio input
function q_joint = motor_position_to_joint( ...
    q_motor, q_motor_ref, q_joint_ref, ...
    motor_sign, motor_ratio)
%#codegen
%
% 电机位置反馈转换为运动学关节角
%
% q_motor      当前电机位置反馈，rad
% q_motor_ref  标定参考姿态下的电机位置，rad
% q_joint_ref  标定参考姿态下的模型关节角，rad
% motor_sign   +1 或 -1
% motor_ratio  电机角变化/关节角变化

qm = single(q_motor);
qm0 = single(q_motor_ref);
qj0 = single(q_joint_ref);
sgn = single(motor_sign);
ratio = single(motor_ratio);

q_joint = qj0;

if abs(ratio) > single(1.0e-6)
    q_joint = qj0 + ...
        sgn * (qm - qm0) / ratio;
end

end

== matlab function testing_DM_hby/FiveBar_FK_Left_Actual ==
  data: x output; alpha input; y output; beta input; L1 input; L2 input; L3 input; L4 input; L5 input; leg_length output; leg_angle output; valid output
function [x, y, leg_length, leg_angle, valid] = ...
    fivebar_fk(alpha, beta, L1, L2, L3, L4, L5)
%#codegen
%
% 平面五连杆正运动学
%
% O = (0,0)
% D = (L5,0)
% x 向右为正
% y 向下为正
%
% 角度单位：rad
% 长度单位：m

x = single(0.0);
y = single(0.0);
leg_length = single(0.0);
leg_angle  = single(0.0);
valid = false;

eps_d = single(1.0e-6);

%% 两根主动杆末端

Ax = L1 * cos(alpha);
Ay = L1 * sin(alpha);

Cx = L5 + L4 * cos(beta);
Cy = L4 * sin(beta);

%% 求以 A、C 为圆心的两个圆交点

dx = Cx - Ax;
dy = Cy - Ay;

Dac = sqrt(dx * dx + dy * dy);

if Dac < eps_d
    return;
end

if Dac > (L2 + L3)
    return;
end

if Dac < abs(L2 - L3)
    return;
end

a = ...
    (L2 * L2 - L3 * L3 + Dac * Dac) / ...
    (single(2.0) * Dac);

h2 = L2 * L2 - a * a;

if h2 < single(-1.0e-7)
    return;
end

if h2 < single(0.0)
    h2 = single(0.0);
end

h = sqrt(h2);

ux = dx / Dac;
uy = dy / Dac;

Mx = Ax + a * ux;
My = Ay + a * uy;

% 两个可能的轮心位置
x1 = Mx - h * uy;
y1 = My + h * ux;

x2 = Mx + h * uy;
y2 = My - h * ux;

% y 向下为正，因此选下面的交点
if y1 >= y2
    x = x1;
    y = y1;
else
    x = x2;
    y = y2;
end

%% 虚拟腿长和虚拟腿角

center_x = L5 / single(2.0);

leg_x = x - center_x;
leg_y = y;

leg_length = sqrt(leg_x * leg_x + leg_y * leg_y);

% 竖直向下时 leg_angle = 0
leg_angle = atan2(leg_x, leg_y);

valid = true;

end

== matlab function testing_DM_hby/FiveBar_FK_Right_Actual ==
  data: x output; alpha input; y output; beta input; L1 input; L2 input; L3 input; L4 input; L5 input; leg_length output; leg_angle output; valid output
function [x, y, leg_length, leg_angle, valid] = ...
    fivebar_fk(alpha, beta, L1, L2, L3, L4, L5)
%#codegen
%
% 平面五连杆正运动学
%
% O = (0,0)
% D = (L5,0)
% x 向右为正
% y 向下为正
%
% 角度单位：rad
% 长度单位：m

x = single(0.0);
y = single(0.0);
leg_length = single(0.0);
leg_angle  = single(0.0);
valid = false;

eps_d = single(1.0e-6);

%% 两根主动杆末端

Ax = L1 * cos(alpha);
Ay = L1 * sin(alpha);

Cx = L5 + L4 * cos(beta);
Cy = L4 * sin(beta);

%% 求以 A、C 为圆心的两个圆交点

dx = Cx - Ax;
dy = Cy - Ay;

Dac = sqrt(dx * dx + dy * dy);

if Dac < eps_d
    return;
end

if Dac > (L2 + L3)
    return;
end

if Dac < abs(L2 - L3)
    return;
end

a = ...
    (L2 * L2 - L3 * L3 + Dac * Dac) / ...
    (single(2.0) * Dac);

h2 = L2 * L2 - a * a;

if h2 < single(-1.0e-7)
    return;
end

if h2 < single(0.0)
    h2 = single(0.0);
end

h = sqrt(h2);

ux = dx / Dac;
uy = dy / Dac;

Mx = Ax + a * ux;
My = Ay + a * uy;

% 两个可能的轮心位置
x1 = Mx - h * uy;
y1 = My + h * ux;

x2 = Mx + h * uy;
y2 = My - h * ux;

% y 向下为正，因此选下面的交点
if y1 >= y2
    x = x1;
    y = y1;
else
    x = x2;
    y = y2;
end

%% 虚拟腿长和虚拟腿角

center_x = L5 / single(2.0);

leg_x = x - center_x;
leg_y = y;

leg_length = sqrt(leg_x * leg_x + leg_y * leg_y);

% 竖直向下时 leg_angle = 0
leg_angle = atan2(leg_x, leg_y);

valid = true;

end

== matlab function testing_DM_hby/FiveBar_Animation_Left_Actual ==
  data: time_in input; alpha input; beta input; xB input; yB input; L1 input; L4 input; L5 input; valid input
function FiveBar_Animation( ...
    time_in, alpha, beta, xB, yB, L1, L4, L5, valid)
%#codegen

coder.extrinsic('fivebar_plot_smooth');

if coder.target('Sfun')

    fivebar_plot_smooth( ...
        double(time_in), ...
        double(alpha), ...
        double(beta), ...
        double(xB), ...
        double(yB), ...
        double(L1), ...
        double(L4), ...
        double(L5), ...
        logical(valid));

end

end

== matlab function testing_DM_hby/Motor_Position_To_Joint ==
  data: q_motor input; q_joint output; qm0 input; qj0 input; motor_sign input; motor_ratio input; valid output
function [q_joint, valid] = Motor_Position_To_Joint( ...
    q_motor, qm0, qj0, motor_sign, motor_ratio)
%#codegen
% 将电机反馈角度转换为五连杆主动关节角
%
% 标定关系：
% q_joint = qj0 + (q_motor - qm0) * motor_sign / motor_ratio

% 统一使用single，匹配ROS消息中的float32
q_motor    = single(q_motor);
qm0        = single(qm0);
qj0        = single(qj0);
motor_sign = single(motor_sign);
motor_ratio = single(motor_ratio);

% 默认输出
q_joint = qj0;
valid = false;

% 检查输入是否有效
if ~isfinite(q_motor) || ...
   ~isfinite(qm0) || ...
   ~isfinite(qj0) || ...
   ~isfinite(motor_sign) || ...
   ~isfinite(motor_ratio)
    return;
end

% 防止除以0
if abs(motor_ratio) < single(1.0e-6)
    return;
end

% 电机角转换为关节角
q_joint = qj0 + ...
    (q_motor - qm0) * motor_sign / motor_ratio;

valid = isfinite(q_joint);

end

== matlab function testing_DM_hby/Motor_Position_To_Joint_LA ==
  data: q_motor input; q_joint output; qm0 input; qj0 input; motor_sign input; motor_ratio input; valid output
function [q_joint, valid] = Motor_Position_To_Joint( ...
    q_motor, qm0, qj0, motor_sign, motor_ratio)
%#codegen
% 将电机反馈角度转换为五连杆主动关节角
%
% 标定关系：
% q_joint = qj0 + (q_motor - qm0) * motor_sign / motor_ratio

% 统一使用single，匹配ROS消息中的float32
q_motor    = single(q_motor);
qm0        = single(qm0);
qj0        = single(qj0);
motor_sign = single(motor_sign);
motor_ratio = single(motor_ratio);

% 默认输出
q_joint = qj0;
valid = false;

% 检查输入是否有效
if ~isfinite(q_motor) || ...
   ~isfinite(qm0) || ...
   ~isfinite(qj0) || ...
   ~isfinite(motor_sign) || ...
   ~isfinite(motor_ratio)
    return;
end

% 防止除以0
if abs(motor_ratio) < single(1.0e-6)
    return;
end

% 电机角转换为关节角
q_joint = qj0 + ...
    (q_motor - qm0) * motor_sign / motor_ratio;

valid = isfinite(q_joint);

end

== matlab function testing_DM_hby/Motor_Position_To_Joint_LB ==
  data: q_motor input; q_joint output; qm0 input; qj0 input; motor_sign input; motor_ratio input; valid output
function [q_joint, valid] = Motor_Position_To_Joint( ...
    q_motor, qm0, qj0, motor_sign, motor_ratio)
%#codegen
% 将电机反馈角度转换为五连杆主动关节角
%
% 标定关系：
% q_joint = qj0 + (q_motor - qm0) * motor_sign / motor_ratio

% 统一使用single，匹配ROS消息中的float32
q_motor    = single(q_motor);
qm0        = single(qm0);
qj0        = single(qj0);
motor_sign = single(motor_sign);
motor_ratio = single(motor_ratio);

% 默认输出
q_joint = qj0;
valid = false;

% 检查输入是否有效
if ~isfinite(q_motor) || ...
   ~isfinite(qm0) || ...
   ~isfinite(qj0) || ...
   ~isfinite(motor_sign) || ...
   ~isfinite(motor_ratio)
    return;
end

% 防止除以0
if abs(motor_ratio) < single(1.0e-6)
    return;
end

% 电机角转换为关节角
q_joint = qj0 + ...
    (q_motor - qm0) * motor_sign / motor_ratio;

valid = isfinite(q_joint);

end

== matlab function testing_DM_hby/FiveBar_FK1 ==
  data: x output; alpha input; y output; beta input; L1 input; L2 input; L3 input; L4 input; L5 input; leg_length output; leg_angle output; valid output
function [x, y, leg_length, leg_angle, valid] = ...
    fivebar_fk(alpha, beta, L1, L2, L3, L4, L5)
%#codegen
%
% 平面五连杆正运动学
%
% O = (0,0)
% D = (L5,0)
% x 向右为正
% y 向下为正
%
% 角度单位：rad
% 长度单位：m

x = single(0.0);
y = single(0.0);
leg_length = single(0.0);
leg_angle  = single(0.0);
valid = false;

eps_d = single(1.0e-6);

%% 两根主动杆末端

Ax = L1 * cos(alpha);
Ay = L1 * sin(alpha);

Cx = L5 + L4 * cos(beta);
Cy = L4 * sin(beta);

%% 求以 A、C 为圆心的两个圆交点

dx = Cx - Ax;
dy = Cy - Ay;

Dac = sqrt(dx * dx + dy * dy);

if Dac < eps_d
    return;
end

if Dac > (L2 + L3)
    return;
end

if Dac < abs(L2 - L3)
    return;
end

a = ...
    (L2 * L2 - L3 * L3 + Dac * Dac) / ...
    (single(2.0) * Dac);

h2 = L2 * L2 - a * a;

if h2 < single(-1.0e-7)
    return;
end

if h2 < single(0.0)
    h2 = single(0.0);
end

h = sqrt(h2);

ux = dx / Dac;
uy = dy / Dac;

Mx = Ax + a * ux;
My = Ay + a * uy;

% 两个可能的轮心位置
x1 = Mx - h * uy;
y1 = My + h * ux;

x2 = Mx + h * uy;
y2 = My - h * ux;

% y 向下为正，因此选下面的交点
if y1 >= y2
    x = x1;
    y = y1;
else
    x = x2;
    y = y2;
end

%% 虚拟腿长和虚拟腿角

center_x = L5 / single(2.0);

leg_x = x - center_x;
leg_y = y;

leg_length = sqrt(leg_x * leg_x + leg_y * leg_y);

% 竖直向下时 leg_angle = 0
leg_angle = atan2(leg_x, leg_y);

valid = true;

end

== matlab function testing_DM_hby/FiveBar_FK ==
  data: x output; alpha input; y output; beta input; L1 input; L2 input; L3 input; L4 input; L5 input; leg_length output; leg_angle output; valid output
function [x, y, leg_length, leg_angle, valid] = ...
    fivebar_fk(alpha, beta, L1, L2, L3, L4, L5)
%#codegen
%
% 平面五连杆正运动学
%
% O = (0,0)
% D = (L5,0)
% x 向右为正
% y 向下为正
%
% 角度单位：rad
% 长度单位：m

x = single(0.0);
y = single(0.0);
leg_length = single(0.0);
leg_angle  = single(0.0);
valid = false;

eps_d = single(1.0e-6);

%% 两根主动杆末端

Ax = L1 * cos(alpha);
Ay = L1 * sin(alpha);

Cx = L5 + L4 * cos(beta);
Cy = L4 * sin(beta);

%% 求以 A、C 为圆心的两个圆交点

dx = Cx - Ax;
dy = Cy - Ay;

Dac = sqrt(dx * dx + dy * dy);

if Dac < eps_d
    return;
end

if Dac > (L2 + L3)
    return;
end

if Dac < abs(L2 - L3)
    return;
end

a = ...
    (L2 * L2 - L3 * L3 + Dac * Dac) / ...
    (single(2.0) * Dac);

h2 = L2 * L2 - a * a;

if h2 < single(-1.0e-7)
    return;
end

if h2 < single(0.0)
    h2 = single(0.0);
end

h = sqrt(h2);

ux = dx / Dac;
uy = dy / Dac;

Mx = Ax + a * ux;
My = Ay + a * uy;

% 两个可能的轮心位置
x1 = Mx - h * uy;
y1 = My + h * ux;

x2 = Mx + h * uy;
y2 = My - h * ux;

% y 向下为正，因此选下面的交点
if y1 >= y2
    x = x1;
    y = y1;
else
    x = x2;
    y = y2;
end

%% 虚拟腿长和虚拟腿角

center_x = L5 / single(2.0);

leg_x = x - center_x;
leg_y = y;

leg_length = sqrt(leg_x * leg_x + leg_y * leg_y);

% 竖直向下时 leg_angle = 0
leg_angle = atan2(leg_x, leg_y);

valid = true;

end

== matlab function testing_DM_hby/Foot_Sine_Trajectory_HW ==
  data: t input; x_cmd output; trajectory_enable input; x_actual input; y_actual input; path_width input; amplitude input; period input; y_cmd output; trajectory_active output
function [x_cmd, y_cmd, trajectory_active] = ...
    Foot_Sine_Trajectory_HW( ...
    t, trajectory_enable, x_actual, y_actual, ...
    path_width, amplitude, period)
%#codegen
% 从真实脚端当前位置开始生成正弦轨迹
%
% 一个period内：
%   前半周期：沿正弦曲线前进
%   后半周期：沿同一条正弦曲线原路返回
%
% 输入：
%   t                 当前仿真时间，单位s
%   trajectory_enable 轨迹使能，boolean或uint8
%   x_actual           当前真实脚端x坐标，单位m
%   y_actual           当前真实脚端y坐标，单位m
%   path_width         正弦轨迹水平方向长度，单位m
%   amplitude          正弦轨迹振幅，单位m
%   period             完成一次去程和回程的总时间，单位s
%
% 输出：
%   x_cmd              目标脚端x坐标，单位m
%   y_cmd              目标脚端y坐标，单位m
%   trajectory_active  轨迹是否正在运行

persistent last_enable
persistent t_start
persistent x_start
persistent y_start

if isempty(last_enable)
    last_enable = false;
    t_start = 0.0;
    x_start = single(0.0);
    y_start = single(0.0);
end

% 统一数据类型
enable = trajectory_enable ~= 0;

x_actual  = single(x_actual);
y_actual  = single(y_actual);
path_width = single(path_width);
amplitude  = single(amplitude);
period     = single(period);

% 默认保持当前真实脚端位置
x_cmd = x_actual;
y_cmd = y_actual;
trajectory_active = false;

%% 未使能：持续跟踪当前脚端位置

if ~enable
    last_enable = false;

    % 为下一次使能准备初始位置
    x_start = x_actual;
    y_start = y_actual;

    return;
end

%% 检查参数

if ~isfinite(x_actual) || ...
   ~isfinite(y_actual) || ...
   ~isfinite(path_width) || ...
   ~isfinite(amplitude) || ...
   ~isfinite(period)
    return;
end

if period <= single(1.0e-3)
    return;
end

%% 检测使能上升沿，记录真实起点

if ~last_enable
    t_start = double(t);
    x_start = x_actual;
    y_start = y_actual;
    last_enable = true;
end

%% 生成往返轨迹

tau = double(t) - t_start;

if tau < 0.0
    tau = 0.0;
end

% 将时间限制在一个周期内，然后重复运动
period_double = double(period);
tau_cycle = mod(tau, period_double);

% s的运动规律：
% t=0          时 s=0
% t=period/2   时 s=1
% t=period     时 s=0
%
% 因此完成一次前进和原路返回
s = 0.5 - 0.5*cos(2.0*pi*tau_cycle/period_double);

% x沿路径方向运动
x_cmd = x_start + path_width*single(s);

% y是x路径参数s的正弦函数
% 去程和回程使用同一个s-y关系，所以会严格原路返回
y_cmd = y_start + ...
    amplitude*sin(single(2.0*pi)*single(s));

trajectory_active = true;

end

== matlab function testing_DM_hby/FiveBar_IK1 ==
  data: x_cmd input; alpha_cmd output; y_cmd input; L1 input; L2 input; L3 input; L4 input; L5 input; alpha_ref input; beta_ref input; beta_cmd output; valid output
function [alpha_cmd, beta_cmd, valid] = fivebar_ik( ...
    x_cmd, y_cmd, L1, L2, L3, L4, L5, ...
    alpha_ref, beta_ref)
%#codegen
%
% 平面五连杆逆运动学
%
% 坐标系：
% 左侧固定关节 O = (0,0)
% 右侧固定关节 D = (L5,0)
% x 向右为正
% y 向下为正
%
% 长度单位：m
% 角度单位：rad

alpha_cmd = alpha_ref;
beta_cmd  = beta_ref;
valid = false;

eps_r = single(1.0e-6);

%% 左侧两连杆

rx1 = x_cmd;
ry1 = y_cmd;

r1 = sqrt(rx1 * rx1 + ry1 * ry1);

if r1 < eps_r
    return;
end

c_alpha = ...
    (r1 * r1 + L1 * L1 - L2 * L2) / ...
    (single(2.0) * L1 * r1);

if c_alpha > single(1.0) || c_alpha < single(-1.0)
    return;
end

c_alpha = min(max(c_alpha, single(-1.0)), single(1.0));

phi1 = atan2(ry1, rx1);
delta1 = acos(c_alpha);

alpha_1 = phi1 + delta1;
alpha_2 = phi1 - delta1;

err_alpha_1 = abs(atan2( ...
    sin(alpha_1 - alpha_ref), ...
    cos(alpha_1 - alpha_ref)));

err_alpha_2 = abs(atan2( ...
    sin(alpha_2 - alpha_ref), ...
    cos(alpha_2 - alpha_ref)));

if err_alpha_1 <= err_alpha_2
    alpha_cmd = alpha_1;
else
    alpha_cmd = alpha_2;
end

%% 右侧两连杆

rx2 = x_cmd - L5;
ry2 = y_cmd;

r2 = sqrt(rx2 * rx2 + ry2 * ry2);

if r2 < eps_r
    return;
end

c_beta = ...
    (r2 * r2 + L4 * L4 - L3 * L3) / ...
    (single(2.0) * L4 * r2);

if c_beta > single(1.0) || c_beta < single(-1.0)
    return;
end

c_beta = min(max(c_beta, single(-1.0)), single(1.0));

phi2 = atan2(ry2, rx2);
delta2 = acos(c_beta);

beta_1 = phi2 + delta2;
beta_2 = phi2 - delta2;

err_beta_1 = abs(atan2( ...
    sin(beta_1 - beta_ref), ...
    cos(beta_1 - beta_ref)));

err_beta_2 = abs(atan2( ...
    sin(beta_2 - beta_ref), ...
    cos(beta_2 - beta_ref)));

if err_beta_1 <= err_beta_2
    beta_cmd = beta_1;
else
    beta_cmd = beta_2;
end

valid = true;

end

== matlab function testing_DM_hby/Left_Joint_To_Motor_L ==
  data: alpha_cmd input; p_LA_target output; beta_cmd input; p_LB_target output; valid output
function [p_LA_target, p_LB_target, valid] = ...
    Left_Joint_To_Motor(alpha_cmd, beta_cmd)
%#codegen
% 将左腿两个主动关节目标角转换为电机目标角

% LA标定参数
qm0_LA   = single(-0.3408479690551758);
qj0_LA   = single( 3.504545610856599);
sign_LA  = single(-1.0);
ratio_LA = single( 1.0);

% LB标定参数
qm0_LB   = single(-0.6292438507080078);
qj0_LB   = single( 0.8999130837716534);
sign_LB  = single(-1.0);
ratio_LB = single( 1.0);

alpha_cmd = single(alpha_cmd);
beta_cmd  = single(beta_cmd);

p_LA_target = qm0_LA + ...
    (alpha_cmd - qj0_LA) * ratio_LA / sign_LA;

p_LB_target = qm0_LB + ...
    (beta_cmd - qj0_LB) * ratio_LB / sign_LB;

valid = ...
    isfinite(p_LA_target) && ...
    isfinite(p_LB_target);

end

== matlab function testing_DM_hby/Motor_Target_Velocity_LA ==
  data: p_cmd input; v_des output; enable input; Ts input; cutoff_hz input; max_velocity input; valid output
function [v_des, valid] = Motor_Target_Velocity( ...
    p_cmd, enable, Ts, cutoff_hz, max_velocity)
%#codegen
% 根据最终电机位置目标计算速度目标
%
% p_cmd        最终发送的电机目标位置，rad
% enable       控制使能
% Ts           控制周期，s
% cutoff_hz    速度低通滤波截止频率，Hz
% max_velocity 目标速度限制，rad/s

persistent p_previous
persistent v_previous
persistent was_enabled

if isempty(p_previous)
    p_previous = single(0);
    v_previous = single(0);
    was_enabled = false;
end

p_cmd        = single(p_cmd);
Ts           = single(Ts);
cutoff_hz    = single(cutoff_hz);
max_velocity = single(max_velocity);

v_des = single(0);
valid = false;

control_enabled = enable ~= 0;

if ~control_enabled
    p_previous = p_cmd;
    v_previous = single(0);
    was_enabled = false;
    return;
end

if ~isfinite(p_cmd) || ...
   ~isfinite(Ts) || ...
   ~isfinite(cutoff_hz) || ...
   ~isfinite(max_velocity)
    return;
end

if Ts <= single(1.0e-6)
    return;
end

% 刚使能时避免产生巨大差分速度
if ~was_enabled
    p_previous = p_cmd;
    v_previous = single(0);
    was_enabled = true;

    v_des = single(0);
    valid = true;
    return;
end

% 原始差分速度
v_raw = (p_cmd - p_previous) / Ts;

% 速度限幅
v_raw = min(max(v_raw, -max_velocity), max_velocity);

% 一阶低通滤波
if cutoff_hz > single(0)
    filter_coefficient = ...
        exp(-single(2.0*pi) * cutoff_hz * Ts);

    v_des = ...
        filter_coefficient * v_previous + ...
        (single(1.0) - filter_coefficient) * v_raw;
else
    v_des = v_raw;
end

% 再做一次限幅
v_des = min(max(v_des, -max_velocity), max_velocity);

p_previous = p_cmd;
v_previous = v_des;

valid = isfinite(v_des);

end

== matlab function testing_DM_hby/Motor_Target_Velocity_LB ==
  data: p_cmd input; v_des output; enable input; Ts input; cutoff_hz input; max_velocity input; valid output
function [v_des, valid] = Motor_Target_Velocity( ...
    p_cmd, enable, Ts, cutoff_hz, max_velocity)
%#codegen
% 根据最终电机位置目标计算速度目标
%
% p_cmd        最终发送的电机目标位置，rad
% enable       控制使能
% Ts           控制周期，s
% cutoff_hz    速度低通滤波截止频率，Hz
% max_velocity 目标速度限制，rad/s

persistent p_previous
persistent v_previous
persistent was_enabled

if isempty(p_previous)
    p_previous = single(0);
    v_previous = single(0);
    was_enabled = false;
end

p_cmd        = single(p_cmd);
Ts           = single(Ts);
cutoff_hz    = single(cutoff_hz);
max_velocity = single(max_velocity);

v_des = single(0);
valid = false;

control_enabled = enable ~= 0;

if ~control_enabled
    p_previous = p_cmd;
    v_previous = single(0);
    was_enabled = false;
    return;
end

if ~isfinite(p_cmd) || ...
   ~isfinite(Ts) || ...
   ~isfinite(cutoff_hz) || ...
   ~isfinite(max_velocity)
    return;
end

if Ts <= single(1.0e-6)
    return;
end

% 刚使能时避免产生巨大差分速度
if ~was_enabled
    p_previous = p_cmd;
    v_previous = single(0);
    was_enabled = true;

    v_des = single(0);
    valid = true;
    return;
end

% 原始差分速度
v_raw = (p_cmd - p_previous) / Ts;

% 速度限幅
v_raw = min(max(v_raw, -max_velocity), max_velocity);

% 一阶低通滤波
if cutoff_hz > single(0)
    filter_coefficient = ...
        exp(-single(2.0*pi) * cutoff_hz * Ts);

    v_des = ...
        filter_coefficient * v_previous + ...
        (single(1.0) - filter_coefficient) * v_raw;
else
    v_des = v_raw;
end

% 再做一次限幅
v_des = min(max(v_des, -max_velocity), max_velocity);

p_previous = p_cmd;
v_previous = v_des;

valid = isfinite(v_des);

end

== matlab function testing_DM_hby/FiveBar_Animation_Compare ==
  data: alpha_actual input; dummy output; beta_actual input; x_actual input; y_actual input; x_cmd input; y_cmd input; phase input; x_home input; y_home input; path_width input; amplitude input; L1 input; L2 input; L3 input; L4 input; L5 input
function dummy = FiveBar_Animation_Compare( ...
    alpha_actual, beta_actual, ...
    x_actual, y_actual, ...
    x_cmd, y_cmd, ...
    phase, ...
    x_home, y_home, ...
    path_width, amplitude, ...
    L1, L2, L3, L4, L5)
%#codegen
%
% phase = 0：关闭
% phase = 1：正在回到正弦起点
% phase = 2：正在执行正弦轨迹

coder.extrinsic('fivebar_animation_compare_plot');

dummy = uint8(0);

if coder.target('MATLAB') || coder.target('Sfun')

    fivebar_animation_compare_plot( ...
        double(alpha_actual), ...
        double(beta_actual), ...
        double(x_actual), ...
        double(y_actual), ...
        double(x_cmd), ...
        double(y_cmd), ...
        uint8(phase), ...
        double(x_home), ...
        double(y_home), ...
        double(path_width), ...
        double(amplitude), ...
        double(L1), ...
        double(L2), ...
        double(L3), ...
        double(L4), ...
        double(L5));
end

end
